simulink model "downblockDiagram"  (Simulink 7.7)
settings: Solver=ode5  StartTime=0.0  StopTime=10.0  FixedStep=0.0005  RelTol=1e-3
undefined symbols (not defined in the file): ba, bt, g, I1zt, Ix2, Ixz2, Iy2, Iz2, K1, K2, K3, K4, Ka, Kt, l1, l2c, m2, tau
settings Model: Creator=jrpeterson  LastModifiedBy=jrpeterson
settings HardwareCC: ProdBitPerInt=16  ProdBitPerPointer=8  ProdIntDivRoundTo=Zero  ProdWordSize=8  ProdShiftRightIntArith=off  ProdHWDeviceType=Intel->8051 Compatible

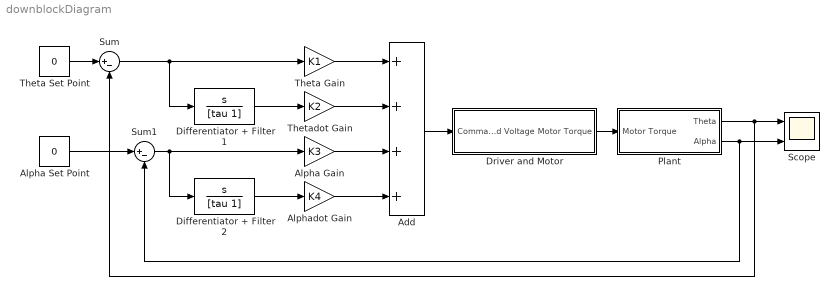
== system downblockDiagram ==
  Add : Sum  Inputs=++++
  Alpha Gain : Gain  Gain=K3
  Alpha Set Point : Constant  Value=0
  Alphadot Gain : Gain  Gain=K4
  Differentiator + Filter 1 : TransferFcn  Numerator=[1 0]  Denominator=[tau 1]
  Differentiator + Filter 2 : TransferFcn  Numerator=[1 0]  Denominator=[tau 1]
  Driver and Motor : Subsystem
  Plant : Subsystem
  Scope : Scope  NumInputPorts=2
      settings: YMin=-5~-5  YMax=5~5
  Sum : Sum  Inputs=|+-
  Sum1 : Sum  Inputs=|+-
  Theta Gain : Gain  Gain=K1
  Theta Set Point : Constant  Value=0
  Thetadot Gain : Gain  Gain=K2
  wires:
  Theta Gain/1 -> Add/1
  Thetadot Gain/1 -> Add/2
  Alpha Gain/1 -> Add/3
  Alphadot Gain/1 -> Add/4
  Add/1 -> Driver and Motor/1(Command Voltage)
  Driver and Motor/1(Motor Torque) -> Plant/1(Motor Torque)
  Theta Set Point/1 -> Sum/1
  Sum/1 -> Theta Gain/1, Differentiator + Filter 1/1
  Plant/1(Theta) -> Sum/2, Scope/1
  Alpha Set Point/1 -> Sum1/1
  Plant/2(Alpha) -> Sum1/2, Scope/2
  Sum1/1 -> Alpha Gain/1, Differentiator + Filter 2/1
  Differentiator + Filter 1/1 -> Thetadot Gain/1
  Differentiator + Filter 2/1 -> Alphadot Gain/1

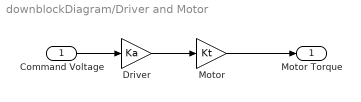
== system downblockDiagram/Driver and Motor ==
  Command Voltage : Inport
  Driver : Gain  Gain=Ka
  "Motor " : Gain  Gain=Kt
  Motor Torque : Outport
  wires:
  Command Voltage/1 -> Driver/1
  Driver/1 -> "Motor "/1
  "Motor "/1 -> Motor Torque/1

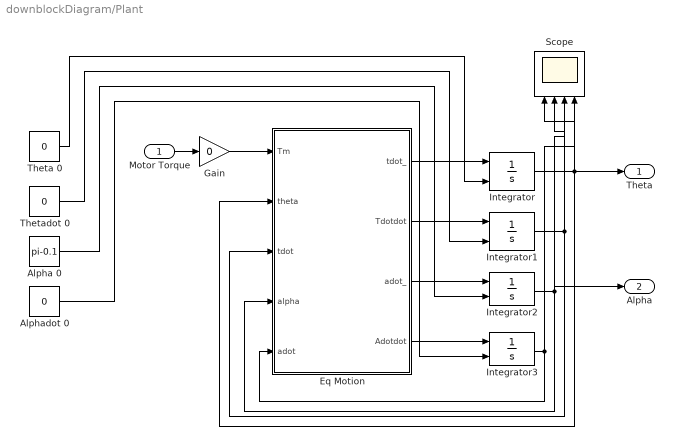
== system downblockDiagram/Plant ==
  Motor Torque : Inport
  Alpha 0 : Constant  Value=pi-0.1
  Alphadot 0 : Constant  Value=0
  Eq Motion : Stateflow chart  TreatAsAtomicUnit=on
  Gain : Gain  Gain=0
  Integrator{,1..3} (4 alike) : Integrator  InitialConditionSource=external
  Scope : Scope  NumInputPorts=4
      settings: YMin=-5~-5~-5~-5  YMax=5~5~5~5  SaveName=LinearSystemResponse
  Theta 0 : Constant  Value=0
  Thetadot 0 : Constant  Value=0
  Theta : Outport
  Alpha : Outport  Port=2
  wires:
  Motor Torque/1 -> Gain/1
  Eq Motion/1(tdot_) -> Integrator/1
  Eq Motion/2(Tdotdot) -> Integrator1/1
  Eq Motion/3(adot_) -> Integrator2/1
  Eq Motion/4(Adotdot) -> Integrator3/1
  Integrator3/1 -> Eq Motion/5(adot), Scope/4
  Integrator2/1 -> Eq Motion/4(alpha), Alpha/1, Scope/3
  Integrator1/1 -> Eq Motion/3(tdot), Scope/2
  Integrator/1 -> Eq Motion/2(theta), Scope/1, Theta/1
  Theta 0/1 -> Integrator/2
  Thetadot 0/1 -> Integrator1/2
  Alpha 0/1 -> Integrator2/2
  Alphadot 0/1 -> Integrator3/2
  Gain/1 -> Eq Motion/1(Tm)

== matlab function Plant/Eq Motion ==
  data: Tm input double; tdot_ output double; theta input double; tdot input double; alpha input double; adot input double; m2 parameter double; I1zt parameter double; Ix2 parameter double; Iy2 parameter double; Iz2 parameter double; Ixz2 parameter double; g parameter double; l1 parameter double; l2c parameter double; ba parameter double; bt parameter double; Tdotdot output double; adot_ output double; Adotdot output double
function [tdot_, Tdotdot, adot_, Adotdot] = eqMotionLinear(Tm, theta,tdot,alpha,adot, m2, I1zt, Ix2, Iy2, Iz2, Ixz2, g, l1, l2c, ba, bt)
% we currently assume differential coulomb friction and damping for theta,
% but not for alpha
% linearized about alpha = pi, theta = 0
tdot_ = tdot;
adot_ = adot;

%%%%%%%%%%%%
% Linear Damping

% Neglect Friction

C1 = Iz2+m2*l2c*l2c;  C2 = Iy2+m2*l2c*l2c;   C3 = m2*l1*l2c-Ixz2;  C4 = l2c*m2*g;

C7 = (I1zt + C2*(pi*pi - 2*pi*alpha) + Ix2 + m2*l1*l1)*C1 - C3*C3;

Tdotdot = (1/C7)*(C3*C4*(alpha - pi) - C3*ba*adot - C1*bt*tdot + C1*Tm);

Adotdot = (1/C1)*(Tdotdot*C3 + C4*pi - C4*alpha - ba*adot);
end
